simulink model "ResearchPaper4Fig8"  (R2015b)
settings: Solver=VariableStepAuto  StartTime=0.0  StopTime=10.0  RelTol=1e-3
libraries: xbsIndex_r4 x484, commfilt2 x1, commrandsrc3 x1, commdigbbndam3 x1
(part 3 of 3)

== system ResearchPaper4Fig8/Conventional RVTDNN6/Hidden Neuron4/Weight Update3 for H.N ==
  eta'grad : Inport
  xin1 : Inport  Port=2
  AddSub : xbsIndex_r4/AddSub  mode=Addition  use_carryin=off  use_carryout=off  en=off  latency=0  precision=Full  arith_type=Unsigned  n_bits=16  bin_pt=14  quantization=Truncate  overflow=Wrap  use_behavioral_HDL=off  hw_selection=Fabric  pipelined=off  dbl_ovrd=off  block_type=addsub
  Mult : xbsIndex_r4/Mult  precision=Full  arith_type="Signed  (2's comp)"  n_bits=16  bin_pt=14  quantization=Truncate  overflow=Wrap  en=off  latency=0  use_behavioral_HDL=off  opt=Speed  use_embedded=on  optimum_pipeline=off  pipeline=on  dbl_ovrd=off  use_rpm=on  placement_style=Triangular  block_type=mult
  Register : xbsIndex_r4/Register  init=0  rst=off  en=off  dbl_ovrd=off  block_type=register
  w11 : Outport
  wires:
  Mult/1 -> AddSub/1
  Register/1 -> w11/1, AddSub/2
  AddSub/1 -> Register/1
  eta'grad/1 -> Mult/1
  xin1/1 -> Mult/2

== system ResearchPaper4Fig8/Conventional RVTDNN6/Hidden Neuron4/Weight Update4 for H.N ==
  eta'grad : Inport
  xin1 : Inport  Port=2
  AddSub : xbsIndex_r4/AddSub  mode=Addition  use_carryin=off  use_carryout=off  en=off  latency=0  precision=Full  arith_type=Unsigned  n_bits=16  bin_pt=14  quantization=Truncate  overflow=Wrap  use_behavioral_HDL=off  hw_selection=Fabric  pipelined=off  dbl_ovrd=off  block_type=addsub
  Mult : xbsIndex_r4/Mult  precision=Full  arith_type="Signed  (2's comp)"  n_bits=16  bin_pt=14  quantization=Truncate  overflow=Wrap  en=off  latency=0  use_behavioral_HDL=off  opt=Speed  use_embedded=on  optimum_pipeline=off  pipeline=on  dbl_ovrd=off  use_rpm=on  placement_style=Triangular  block_type=mult
  Register : xbsIndex_r4/Register  init=0  rst=off  en=off  dbl_ovrd=off  block_type=register
  w11 : Outport
  wires:
  Mult/1 -> AddSub/1
  Register/1 -> w11/1, AddSub/2
  AddSub/1 -> Register/1
  eta'grad/1 -> Mult/1
  xin1/1 -> Mult/2

== system ResearchPaper4Fig8/Conventional RVTDNN6/Hidden Neuron4/Weight Update5 for H.N ==
  eta'grad : Inport
  xin1 : Inport  Port=2
  AddSub : xbsIndex_r4/AddSub  mode=Addition  use_carryin=off  use_carryout=off  en=off  latency=0  precision=Full  arith_type=Unsigned  n_bits=16  bin_pt=14  quantization=Truncate  overflow=Wrap  use_behavioral_HDL=off  hw_selection=Fabric  pipelined=off  dbl_ovrd=off  block_type=addsub
  Mult : xbsIndex_r4/Mult  precision=Full  arith_type="Signed  (2's comp)"  n_bits=16  bin_pt=14  quantization=Truncate  overflow=Wrap  en=off  latency=0  use_behavioral_HDL=off  opt=Speed  use_embedded=on  optimum_pipeline=off  pipeline=on  dbl_ovrd=off  use_rpm=on  placement_style=Triangular  block_type=mult
  Register : xbsIndex_r4/Register  init=0  rst=off  en=off  dbl_ovrd=off  block_type=register
  w11 : Outport
  wires:
  Mult/1 -> AddSub/1
  Register/1 -> w11/1, AddSub/2
  AddSub/1 -> Register/1
  eta'grad/1 -> Mult/1
  xin1/1 -> Mult/2

== system ResearchPaper4Fig8/Conventional RVTDNN6/Hidden Neuron4/Weight Update6 for H.N ==
  eta'grad : Inport
  xin1 : Inport  Port=2
  AddSub : xbsIndex_r4/AddSub  mode=Addition  use_carryin=off  use_carryout=off  en=off  latency=0  precision=Full  arith_type=Unsigned  n_bits=16  bin_pt=14  quantization=Truncate  overflow=Wrap  use_behavioral_HDL=off  hw_selection=Fabric  pipelined=off  dbl_ovrd=off  block_type=addsub
  Mult : xbsIndex_r4/Mult  precision=Full  arith_type="Signed  (2's comp)"  n_bits=16  bin_pt=14  quantization=Truncate  overflow=Wrap  en=off  latency=0  use_behavioral_HDL=off  opt=Speed  use_embedded=on  optimum_pipeline=off  pipeline=on  dbl_ovrd=off  use_rpm=on  placement_style=Triangular  block_type=mult
  Register : xbsIndex_r4/Register  init=0  rst=off  en=off  dbl_ovrd=off  block_type=register
  w11 : Outport
  wires:
  Mult/1 -> AddSub/1
  Register/1 -> w11/1, AddSub/2
  AddSub/1 -> Register/1
  eta'grad/1 -> Mult/1
  xin1/1 -> Mult/2

== system ResearchPaper4Fig8/Conventional RVTDNN6/Hidden Neuron5/Bias Update for H.N ==
  eta'grad : Inport
  AddSub : xbsIndex_r4/AddSub  mode=Addition  use_carryin=off  use_carryout=off  en=off  latency=0  precision=Full  arith_type=Unsigned  n_bits=16  bin_pt=14  quantization=Truncate  overflow=Wrap  use_behavioral_HDL=off  hw_selection=Fabric  pipelined=off  dbl_ovrd=off  block_type=addsub
  Register : xbsIndex_r4/Register  init=0  rst=off  en=off  dbl_ovrd=off  block_type=register
  w10 : Outport
  wires:
  Register/1 -> w10/1, AddSub/2
  AddSub/1 -> Register/1
  eta'grad/1 -> AddSub/1

== system ResearchPaper4Fig8/Conventional RVTDNN6/Hidden Neuron5/Hyperbolic Tangent ==
  In1 : Inport
  Constant : xbsIndex_r4/Constant  const=0.0  gui_display_data_type=Fixed-point  arith_type=Signed (2's comp)  n_bits=16  bin_pt=14  preci_type=Single  exp_width=8  frac_width=24  explicit_period=off  period=1  equ=P=C  opselect=C  inp2=PCIN>>17  opr=+  inp1=P  carry=CIN  dbl_ovrd=off  block_type=constant
  Mux : xbsIndex_r4/Mux  inputs=2  en=off  latency=0  precision=Full  arith_type=Unsigned  n_bits=16  bin_pt=14  quantization=Truncate  overflow=Wrap  dbl_ovrd=off  block_type=mux
  Mux1 : xbsIndex_r4/Mux  inputs=2  en=off  latency=0  precision=Full  arith_type=Unsigned  n_bits=16  bin_pt=14  quantization=Truncate  overflow=Wrap  dbl_ovrd=off  block_type=mux
  Negate : xbsIndex_r4/Negate  precision=Full  arith_type=Unsigned  n_bits=16  bin_pt=14  quantization=Truncate  overflow=Wrap  en=off  latency=0  dbl_ovrd=off  block_type=negate
  Negate1 : xbsIndex_r4/Negate  precision=Full  arith_type=Unsigned  n_bits=16  bin_pt=14  quantization=Truncate  overflow=Wrap  en=off  latency=0  dbl_ovrd=off  block_type=negate
  ROM : xbsIndex_r4/ROM  depth=16  initVector=sin(pi*(0:15)/16)  distributed_mem=Distributed memory  rst=off  init_reg=0  en=off  latency=0  gui_display_data_type=Fixed-point  arith_type="Signed  (2's comp)"  n_bits=16  bin_pt=14  preci_type=Single  exp_width=8  frac_width=24  optimize=Area  use_rpm=on  dbl_ovrd=off  block_type=sprom
  Relational : xbsIndex_r4/Relational  mode=a>b  op_type=Bool  en=off  latency=0  dbl_ovrd=off  block_type=relational
  Shift : xbsIndex_r4/Shift  shift_dir=Left  shift_bits=13  en=off  latency=0  precision=Full  arith_type="Signed  (2's comp)"  n_bits=16  bin_pt=14  quantization=Truncate  overflow=Wrap  dbl_ovrd=off  block_type=shift
  Out1 : Outport
  wires:
  Relational/1 -> Mux1/1, Mux/1
  Mux/1 -> Shift/1
  Mux1/1 -> Out1/1
  ROM/1 -> Negate1/1, Mux1/2
  Negate1/1 -> Mux1/3
  Constant/1 -> Relational/1
  In1/1 -> Negate/1, Relational/2, Mux/2
  Negate/1 -> Mux/3
  Shift/1 -> ROM/1

== system ResearchPaper4Fig8/Conventional RVTDNN6/Hidden Neuron5/Sum ==
  In1 : Inport
  In2 : Inport  Port=2
  In3 : Inport  Port=3
  In4 : Inport  Port=4
  In5 : Inport  Port=5
  In6 : Inport  Port=6
  In7 : Inport  Port=7
  AddSub{,1..5} (6 alike) : xbsIndex_r4/AddSub  mode=Addition  use_carryin=off  use_carryout=off  en=off  latency=0  precision=Full  arith_type=Unsigned  n_bits=16  bin_pt=14  quantization=Truncate  overflow=Wrap  use_behavioral_HDL=off  hw_selection=Fabric  pipelined=off  dbl_ovrd=off  block_type=addsub
  Out : Outport
  wires:
  AddSub4/1 -> AddSub5/2
  AddSub3/1 -> AddSub5/1
  In7/1 -> AddSub4/2
  AddSub1/1 -> AddSub3/2
  AddSub2/1 -> AddSub4/1
  In1/1 -> AddSub/1
  In6/1 -> AddSub2/2
  In2/1 -> AddSub/2
  In4/1 -> AddSub1/2
  AddSub/1 -> AddSub3/1
  In5/1 -> AddSub2/1
  AddSub5/1 -> Out/1
  In3/1 -> AddSub1/1

== system ResearchPaper4Fig8/Conventional RVTDNN6/Hidden Neuron5/Weight Update1 for H.N ==
  eta'grad : Inport
  xin1 : Inport  Port=2
  AddSub : xbsIndex_r4/AddSub  mode=Addition  use_carryin=off  use_carryout=off  en=off  latency=0  precision=Full  arith_type=Unsigned  n_bits=16  bin_pt=14  quantization=Truncate  overflow=Wrap  use_behavioral_HDL=off  hw_selection=Fabric  pipelined=off  dbl_ovrd=off  block_type=addsub
  Mult : xbsIndex_r4/Mult  precision=Full  arith_type="Signed  (2's comp)"  n_bits=16  bin_pt=14  quantization=Truncate  overflow=Wrap  en=off  latency=0  use_behavioral_HDL=off  opt=Speed  use_embedded=on  optimum_pipeline=off  pipeline=on  dbl_ovrd=off  use_rpm=on  placement_style=Triangular  block_type=mult
  Register : xbsIndex_r4/Register  init=0  rst=off  en=off  dbl_ovrd=off  block_type=register
  w11 : Outport
  wires:
  Mult/1 -> AddSub/1
  Register/1 -> w11/1, AddSub/2
  AddSub/1 -> Register/1
  eta'grad/1 -> Mult/1
  xin1/1 -> Mult/2

== system ResearchPaper4Fig8/Conventional RVTDNN6/Hidden Neuron5/Weight Update2 for H.N ==
  eta'grad : Inport
  xin1 : Inport  Port=2
  AddSub : xbsIndex_r4/AddSub  mode=Addition  use_carryin=off  use_carryout=off  en=off  latency=0  precision=Full  arith_type=Unsigned  n_bits=16  bin_pt=14  quantization=Truncate  overflow=Wrap  use_behavioral_HDL=off  hw_selection=Fabric  pipelined=off  dbl_ovrd=off  block_type=addsub
  Mult : xbsIndex_r4/Mult  precision=Full  arith_type="Signed  (2's comp)"  n_bits=16  bin_pt=14  quantization=Truncate  overflow=Wrap  en=off  latency=0  use_behavioral_HDL=off  opt=Speed  use_embedded=on  optimum_pipeline=off  pipeline=on  dbl_ovrd=off  use_rpm=on  placement_style=Triangular  block_type=mult
  Register : xbsIndex_r4/Register  init=0  rst=off  en=off  dbl_ovrd=off  block_type=register
  w11 : Outport
  wires:
  Mult/1 -> AddSub/1
  Register/1 -> w11/1, AddSub/2
  AddSub/1 -> Register/1
  eta'grad/1 -> Mult/1
  xin1/1 -> Mult/2

== system ResearchPaper4Fig8/Conventional RVTDNN6/Hidden Neuron5/Weight Update3 for H.N ==
  eta'grad : Inport
  xin1 : Inport  Port=2
  AddSub : xbsIndex_r4/AddSub  mode=Addition  use_carryin=off  use_carryout=off  en=off  latency=0  precision=Full  arith_type=Unsigned  n_bits=16  bin_pt=14  quantization=Truncate  overflow=Wrap  use_behavioral_HDL=off  hw_selection=Fabric  pipelined=off  dbl_ovrd=off  block_type=addsub
  Mult : xbsIndex_r4/Mult  precision=Full  arith_type="Signed  (2's comp)"  n_bits=16  bin_pt=14  quantization=Truncate  overflow=Wrap  en=off  latency=0  use_behavioral_HDL=off  opt=Speed  use_embedded=on  optimum_pipeline=off  pipeline=on  dbl_ovrd=off  use_rpm=on  placement_style=Triangular  block_type=mult
  Register : xbsIndex_r4/Register  init=0  rst=off  en=off  dbl_ovrd=off  block_type=register
  w11 : Outport
  wires:
  Mult/1 -> AddSub/1
  Register/1 -> w11/1, AddSub/2
  AddSub/1 -> Register/1
  eta'grad/1 -> Mult/1
  xin1/1 -> Mult/2

== system ResearchPaper4Fig8/Conventional RVTDNN6/Hidden Neuron5/Weight Update4 for H.N ==
  eta'grad : Inport
  xin1 : Inport  Port=2
  AddSub : xbsIndex_r4/AddSub  mode=Addition  use_carryin=off  use_carryout=off  en=off  latency=0  precision=Full  arith_type=Unsigned  n_bits=16  bin_pt=14  quantization=Truncate  overflow=Wrap  use_behavioral_HDL=off  hw_selection=Fabric  pipelined=off  dbl_ovrd=off  block_type=addsub
  Mult : xbsIndex_r4/Mult  precision=Full  arith_type="Signed  (2's comp)"  n_bits=16  bin_pt=14  quantization=Truncate  overflow=Wrap  en=off  latency=0  use_behavioral_HDL=off  opt=Speed  use_embedded=on  optimum_pipeline=off  pipeline=on  dbl_ovrd=off  use_rpm=on  placement_style=Triangular  block_type=mult
  Register : xbsIndex_r4/Register  init=0  rst=off  en=off  dbl_ovrd=off  block_type=register
  w11 : Outport
  wires:
  Mult/1 -> AddSub/1
  Register/1 -> w11/1, AddSub/2
  AddSub/1 -> Register/1
  eta'grad/1 -> Mult/1
  xin1/1 -> Mult/2

== system ResearchPaper4Fig8/Conventional RVTDNN6/Hidden Neuron5/Weight Update5 for H.N ==
  eta'grad : Inport
  xin1 : Inport  Port=2
  AddSub : xbsIndex_r4/AddSub  mode=Addition  use_carryin=off  use_carryout=off  en=off  latency=0  precision=Full  arith_type=Unsigned  n_bits=16  bin_pt=14  quantization=Truncate  overflow=Wrap  use_behavioral_HDL=off  hw_selection=Fabric  pipelined=off  dbl_ovrd=off  block_type=addsub
  Mult : xbsIndex_r4/Mult  precision=Full  arith_type="Signed  (2's comp)"  n_bits=16  bin_pt=14  quantization=Truncate  overflow=Wrap  en=off  latency=0  use_behavioral_HDL=off  opt=Speed  use_embedded=on  optimum_pipeline=off  pipeline=on  dbl_ovrd=off  use_rpm=on  placement_style=Triangular  block_type=mult
  Register : xbsIndex_r4/Register  init=0  rst=off  en=off  dbl_ovrd=off  block_type=register
  w11 : Outport
  wires:
  Mult/1 -> AddSub/1
  Register/1 -> w11/1, AddSub/2
  AddSub/1 -> Register/1
  eta'grad/1 -> Mult/1
  xin1/1 -> Mult/2

== system ResearchPaper4Fig8/Conventional RVTDNN6/Hidden Neuron5/Weight Update6 for H.N ==
  eta'grad : Inport
  xin1 : Inport  Port=2
  AddSub : xbsIndex_r4/AddSub  mode=Addition  use_carryin=off  use_carryout=off  en=off  latency=0  precision=Full  arith_type=Unsigned  n_bits=16  bin_pt=14  quantization=Truncate  overflow=Wrap  use_behavioral_HDL=off  hw_selection=Fabric  pipelined=off  dbl_ovrd=off  block_type=addsub
  Mult : xbsIndex_r4/Mult  precision=Full  arith_type="Signed  (2's comp)"  n_bits=16  bin_pt=14  quantization=Truncate  overflow=Wrap  en=off  latency=0  use_behavioral_HDL=off  opt=Speed  use_embedded=on  optimum_pipeline=off  pipeline=on  dbl_ovrd=off  use_rpm=on  placement_style=Triangular  block_type=mult
  Register : xbsIndex_r4/Register  init=0  rst=off  en=off  dbl_ovrd=off  block_type=register
  w11 : Outport
  wires:
  Mult/1 -> AddSub/1
  Register/1 -> w11/1, AddSub/2
  AddSub/1 -> Register/1
  eta'grad/1 -> Mult/1
  xin1/1 -> Mult/2

== system ResearchPaper4Fig8/Conventional RVTDNN6/Hidden Neuron6/Bias Update for H.N ==
  eta'grad : Inport
  AddSub : xbsIndex_r4/AddSub  mode=Addition  use_carryin=off  use_carryout=off  en=off  latency=0  precision=Full  arith_type=Unsigned  n_bits=16  bin_pt=14  quantization=Truncate  overflow=Wrap  use_behavioral_HDL=off  hw_selection=Fabric  pipelined=off  dbl_ovrd=off  block_type=addsub
  Register : xbsIndex_r4/Register  init=0  rst=off  en=off  dbl_ovrd=off  block_type=register
  w10 : Outport
  wires:
  Register/1 -> w10/1, AddSub/2
  AddSub/1 -> Register/1
  eta'grad/1 -> AddSub/1

== system ResearchPaper4Fig8/Conventional RVTDNN6/Hidden Neuron6/Hyperbolic Tangent ==
  In1 : Inport
  Constant : xbsIndex_r4/Constant  const=0.0  gui_display_data_type=Fixed-point  arith_type=Signed (2's comp)  n_bits=16  bin_pt=14  preci_type=Single  exp_width=8  frac_width=24  explicit_period=off  period=1  equ=P=C  opselect=C  inp2=PCIN>>17  opr=+  inp1=P  carry=CIN  dbl_ovrd=off  block_type=constant
  Mux : xbsIndex_r4/Mux  inputs=2  en=off  latency=0  precision=Full  arith_type=Unsigned  n_bits=16  bin_pt=14  quantization=Truncate  overflow=Wrap  dbl_ovrd=off  block_type=mux
  Mux1 : xbsIndex_r4/Mux  inputs=2  en=off  latency=0  precision=Full  arith_type=Unsigned  n_bits=16  bin_pt=14  quantization=Truncate  overflow=Wrap  dbl_ovrd=off  block_type=mux
  Negate : xbsIndex_r4/Negate  precision=Full  arith_type=Unsigned  n_bits=16  bin_pt=14  quantization=Truncate  overflow=Wrap  en=off  latency=0  dbl_ovrd=off  block_type=negate
  Negate1 : xbsIndex_r4/Negate  precision=Full  arith_type=Unsigned  n_bits=16  bin_pt=14  quantization=Truncate  overflow=Wrap  en=off  latency=0  dbl_ovrd=off  block_type=negate
  ROM : xbsIndex_r4/ROM  depth=16  initVector=sin(pi*(0:15)/16)  distributed_mem=Distributed memory  rst=off  init_reg=0  en=off  latency=0  gui_display_data_type=Fixed-point  arith_type="Signed  (2's comp)"  n_bits=16  bin_pt=14  preci_type=Single  exp_width=8  frac_width=24  optimize=Area  use_rpm=on  dbl_ovrd=off  block_type=sprom
  Relational : xbsIndex_r4/Relational  mode=a>b  op_type=Bool  en=off  latency=0  dbl_ovrd=off  block_type=relational
  Shift : xbsIndex_r4/Shift  shift_dir=Left  shift_bits=13  en=off  latency=0  precision=Full  arith_type="Signed  (2's comp)"  n_bits=16  bin_pt=14  quantization=Truncate  overflow=Wrap  dbl_ovrd=off  block_type=shift
  Out1 : Outport
  wires:
  Relational/1 -> Mux1/1, Mux/1
  Mux/1 -> Shift/1
  Mux1/1 -> Out1/1
  ROM/1 -> Negate1/1, Mux1/2
  Negate1/1 -> Mux1/3
  Constant/1 -> Relational/1
  In1/1 -> Negate/1, Relational/2, Mux/2
  Negate/1 -> Mux/3
  Shift/1 -> ROM/1

== system ResearchPaper4Fig8/Conventional RVTDNN6/Hidden Neuron6/Sum ==
  In1 : Inport
  In2 : Inport  Port=2
  In3 : Inport  Port=3
  In4 : Inport  Port=4
  In5 : Inport  Port=5
  In6 : Inport  Port=6
  In7 : Inport  Port=7
  AddSub{,1..5} (6 alike) : xbsIndex_r4/AddSub  mode=Addition  use_carryin=off  use_carryout=off  en=off  latency=0  precision=Full  arith_type=Unsigned  n_bits=16  bin_pt=14  quantization=Truncate  overflow=Wrap  use_behavioral_HDL=off  hw_selection=Fabric  pipelined=off  dbl_ovrd=off  block_type=addsub
  Out : Outport
  wires:
  AddSub4/1 -> AddSub5/2
  AddSub3/1 -> AddSub5/1
  In7/1 -> AddSub4/2
  AddSub1/1 -> AddSub3/2
  AddSub2/1 -> AddSub4/1
  In1/1 -> AddSub/1
  In6/1 -> AddSub2/2
  In2/1 -> AddSub/2
  In4/1 -> AddSub1/2
  AddSub/1 -> AddSub3/1
  In5/1 -> AddSub2/1
  AddSub5/1 -> Out/1
  In3/1 -> AddSub1/1

== system ResearchPaper4Fig8/Conventional RVTDNN6/Hidden Neuron6/Weight Update1 for H.N ==
  eta'grad : Inport
  xin1 : Inport  Port=2
  AddSub : xbsIndex_r4/AddSub  mode=Addition  use_carryin=off  use_carryout=off  en=off  latency=0  precision=Full  arith_type=Unsigned  n_bits=16  bin_pt=14  quantization=Truncate  overflow=Wrap  use_behavioral_HDL=off  hw_selection=Fabric  pipelined=off  dbl_ovrd=off  block_type=addsub
  Mult : xbsIndex_r4/Mult  precision=Full  arith_type="Signed  (2's comp)"  n_bits=16  bin_pt=14  quantization=Truncate  overflow=Wrap  en=off  latency=0  use_behavioral_HDL=off  opt=Speed  use_embedded=on  optimum_pipeline=off  pipeline=on  dbl_ovrd=off  use_rpm=on  placement_style=Triangular  block_type=mult
  Register : xbsIndex_r4/Register  init=0  rst=off  en=off  dbl_ovrd=off  block_type=register
  w11 : Outport
  wires:
  Mult/1 -> AddSub/1
  Register/1 -> w11/1, AddSub/2
  AddSub/1 -> Register/1
  eta'grad/1 -> Mult/1
  xin1/1 -> Mult/2

== system ResearchPaper4Fig8/Conventional RVTDNN6/Hidden Neuron6/Weight Update2 for H.N ==
  eta'grad : Inport
  xin1 : Inport  Port=2
  AddSub : xbsIndex_r4/AddSub  mode=Addition  use_carryin=off  use_carryout=off  en=off  latency=0  precision=Full  arith_type=Unsigned  n_bits=16  bin_pt=14  quantization=Truncate  overflow=Wrap  use_behavioral_HDL=off  hw_selection=Fabric  pipelined=off  dbl_ovrd=off  block_type=addsub
  Mult : xbsIndex_r4/Mult  precision=Full  arith_type="Signed  (2's comp)"  n_bits=16  bin_pt=14  quantization=Truncate  overflow=Wrap  en=off  latency=0  use_behavioral_HDL=off  opt=Speed  use_embedded=on  optimum_pipeline=off  pipeline=on  dbl_ovrd=off  use_rpm=on  placement_style=Triangular  block_type=mult
  Register : xbsIndex_r4/Register  init=0  rst=off  en=off  dbl_ovrd=off  block_type=register
  w11 : Outport
  wires:
  Mult/1 -> AddSub/1
  Register/1 -> w11/1, AddSub/2
  AddSub/1 -> Register/1
  eta'grad/1 -> Mult/1
  xin1/1 -> Mult/2

== system ResearchPaper4Fig8/Conventional RVTDNN6/Hidden Neuron6/Weight Update3 for H.N ==
  eta'grad : Inport
  xin1 : Inport  Port=2
  AddSub : xbsIndex_r4/AddSub  mode=Addition  use_carryin=off  use_carryout=off  en=off  latency=0  precision=Full  arith_type=Unsigned  n_bits=16  bin_pt=14  quantization=Truncate  overflow=Wrap  use_behavioral_HDL=off  hw_selection=Fabric  pipelined=off  dbl_ovrd=off  block_type=addsub
  Mult : xbsIndex_r4/Mult  precision=Full  arith_type="Signed  (2's comp)"  n_bits=16  bin_pt=14  quantization=Truncate  overflow=Wrap  en=off  latency=0  use_behavioral_HDL=off  opt=Speed  use_embedded=on  optimum_pipeline=off  pipeline=on  dbl_ovrd=off  use_rpm=on  placement_style=Triangular  block_type=mult
  Register : xbsIndex_r4/Register  init=0  rst=off  en=off  dbl_ovrd=off  block_type=register
  w11 : Outport
  wires:
  Mult/1 -> AddSub/1
  Register/1 -> w11/1, AddSub/2
  AddSub/1 -> Register/1
  eta'grad/1 -> Mult/1
  xin1/1 -> Mult/2

== system ResearchPaper4Fig8/Conventional RVTDNN6/Hidden Neuron6/Weight Update4 for H.N ==
  eta'grad : Inport
  xin1 : Inport  Port=2
  AddSub : xbsIndex_r4/AddSub  mode=Addition  use_carryin=off  use_carryout=off  en=off  latency=0  precision=Full  arith_type=Unsigned  n_bits=16  bin_pt=14  quantization=Truncate  overflow=Wrap  use_behavioral_HDL=off  hw_selection=Fabric  pipelined=off  dbl_ovrd=off  block_type=addsub
  Mult : xbsIndex_r4/Mult  precision=Full  arith_type="Signed  (2's comp)"  n_bits=16  bin_pt=14  quantization=Truncate  overflow=Wrap  en=off  latency=0  use_behavioral_HDL=off  opt=Speed  use_embedded=on  optimum_pipeline=off  pipeline=on  dbl_ovrd=off  use_rpm=on  placement_style=Triangular  block_type=mult
  Register : xbsIndex_r4/Register  init=0  rst=off  en=off  dbl_ovrd=off  block_type=register
  w11 : Outport
  wires:
  Mult/1 -> AddSub/1
  Register/1 -> w11/1, AddSub/2
  AddSub/1 -> Register/1
  eta'grad/1 -> Mult/1
  xin1/1 -> Mult/2

== system ResearchPaper4Fig8/Conventional RVTDNN6/Hidden Neuron6/Weight Update5 for H.N ==
  eta'grad : Inport
  xin1 : Inport  Port=2
  AddSub : xbsIndex_r4/AddSub  mode=Addition  use_carryin=off  use_carryout=off  en=off  latency=0  precision=Full  arith_type=Unsigned  n_bits=16  bin_pt=14  quantization=Truncate  overflow=Wrap  use_behavioral_HDL=off  hw_selection=Fabric  pipelined=off  dbl_ovrd=off  block_type=addsub
  Mult : xbsIndex_r4/Mult  precision=Full  arith_type="Signed  (2's comp)"  n_bits=16  bin_pt=14  quantization=Truncate  overflow=Wrap  en=off  latency=0  use_behavioral_HDL=off  opt=Speed  use_embedded=on  optimum_pipeline=off  pipeline=on  dbl_ovrd=off  use_rpm=on  placement_style=Triangular  block_type=mult
  Register : xbsIndex_r4/Register  init=0  rst=off  en=off  dbl_ovrd=off  block_type=register
  w11 : Outport
  wires:
  Mult/1 -> AddSub/1
  Register/1 -> w11/1, AddSub/2
  AddSub/1 -> Register/1
  eta'grad/1 -> Mult/1
  xin1/1 -> Mult/2

== system ResearchPaper4Fig8/Conventional RVTDNN6/Hidden Neuron6/Weight Update6 for H.N ==
  eta'grad : Inport
  xin1 : Inport  Port=2
  AddSub : xbsIndex_r4/AddSub  mode=Addition  use_carryin=off  use_carryout=off  en=off  latency=0  precision=Full  arith_type=Unsigned  n_bits=16  bin_pt=14  quantization=Truncate  overflow=Wrap  use_behavioral_HDL=off  hw_selection=Fabric  pipelined=off  dbl_ovrd=off  block_type=addsub
  Mult : xbsIndex_r4/Mult  precision=Full  arith_type="Signed  (2's comp)"  n_bits=16  bin_pt=14  quantization=Truncate  overflow=Wrap  en=off  latency=0  use_behavioral_HDL=off  opt=Speed  use_embedded=on  optimum_pipeline=off  pipeline=on  dbl_ovrd=off  use_rpm=on  placement_style=Triangular  block_type=mult
  Register : xbsIndex_r4/Register  init=0  rst=off  en=off  dbl_ovrd=off  block_type=register
  w11 : Outport
  wires:
  Mult/1 -> AddSub/1
  Register/1 -> w11/1, AddSub/2
  AddSub/1 -> Register/1
  eta'grad/1 -> Mult/1
  xin1/1 -> Mult/2

== system ResearchPaper4Fig8/Conventional RVTDNN6/Output Neuron1/Bias Update for O.N ==
  grad : Inport
  AddSub : xbsIndex_r4/AddSub  mode=Addition  use_carryin=off  use_carryout=off  en=off  latency=0  precision=Full  arith_type=Unsigned  n_bits=16  bin_pt=14  quantization=Truncate  overflow=Wrap  use_behavioral_HDL=off  hw_selection=Fabric  pipelined=off  dbl_ovrd=off  block_type=addsub
  Register : xbsIndex_r4/Register  init=0  rst=off  en=off  dbl_ovrd=off  block_type=register
  w10 : Outport
  wires:
  Register/1 -> w10/1, AddSub/2
  AddSub/1 -> Register/1
  grad/1 -> AddSub/1

== system ResearchPaper4Fig8/Conventional RVTDNN6/Output Neuron1/Sum ==
  In1 : Inport
  In2 : Inport  Port=2
  In3 : Inport  Port=3
  In4 : Inport  Port=4
  In5 : Inport  Port=5
  In6 : Inport  Port=6
  In7 : Inport  Port=7
  AddSub{,1..5} (6 alike) : xbsIndex_r4/AddSub  mode=Addition  use_carryin=off  use_carryout=off  en=off  latency=0  precision=Full  arith_type=Unsigned  n_bits=16  bin_pt=14  quantization=Truncate  overflow=Wrap  use_behavioral_HDL=off  hw_selection=Fabric  pipelined=off  dbl_ovrd=off  block_type=addsub
  Out : Outport
  wires:
  AddSub4/1 -> AddSub5/2
  AddSub3/1 -> AddSub5/1
  In7/1 -> AddSub4/2
  AddSub1/1 -> AddSub3/2
  AddSub2/1 -> AddSub4/1
  In1/1 -> AddSub/1
  In6/1 -> AddSub2/2
  In2/1 -> AddSub/2
  In4/1 -> AddSub1/2
  AddSub/1 -> AddSub3/1
  In5/1 -> AddSub2/1
  AddSub5/1 -> Out/1
  In3/1 -> AddSub1/1

== system ResearchPaper4Fig8/Conventional RVTDNN6/Output Neuron1/Weight Update1 for O.N ==
  eta'grad : Inport
  o1 : Inport  Port=2
  AddSub : xbsIndex_r4/AddSub  mode=Addition  use_carryin=off  use_carryout=off  en=off  latency=0  precision=Full  arith_type=Unsigned  n_bits=16  bin_pt=14  quantization=Truncate  overflow=Wrap  use_behavioral_HDL=off  hw_selection=Fabric  pipelined=off  dbl_ovrd=off  block_type=addsub
  Mult : xbsIndex_r4/Mult  precision=Full  arith_type="Signed  (2's comp)"  n_bits=16  bin_pt=14  quantization=Truncate  overflow=Wrap  en=off  latency=0  use_behavioral_HDL=off  opt=Speed  use_embedded=on  optimum_pipeline=off  pipeline=on  dbl_ovrd=off  use_rpm=on  placement_style=Triangular  block_type=mult
  Register : xbsIndex_r4/Register  init=0  rst=off  en=off  dbl_ovrd=off  block_type=register
  w11 : Outport
  wires:
  Mult/1 -> AddSub/1
  Register/1 -> w11/1, AddSub/2
  AddSub/1 -> Register/1
  eta'grad/1 -> Mult/1
  o1/1 -> Mult/2

== system ResearchPaper4Fig8/Conventional RVTDNN6/Output Neuron1/Weight Update2 for O.N ==
  eta'grad : Inport
  o1 : Inport  Port=2
  AddSub : xbsIndex_r4/AddSub  mode=Addition  use_carryin=off  use_carryout=off  en=off  latency=0  precision=Full  arith_type=Unsigned  n_bits=16  bin_pt=14  quantization=Truncate  overflow=Wrap  use_behavioral_HDL=off  hw_selection=Fabric  pipelined=off  dbl_ovrd=off  block_type=addsub
  Mult : xbsIndex_r4/Mult  precision=Full  arith_type="Signed  (2's comp)"  n_bits=16  bin_pt=14  quantization=Truncate  overflow=Wrap  en=off  latency=0  use_behavioral_HDL=off  opt=Speed  use_embedded=on  optimum_pipeline=off  pipeline=on  dbl_ovrd=off  use_rpm=on  placement_style=Triangular  block_type=mult
  Register : xbsIndex_r4/Register  init=0  rst=off  en=off  dbl_ovrd=off  block_type=register
  w11 : Outport
  wires:
  Mult/1 -> AddSub/1
  Register/1 -> w11/1, AddSub/2
  AddSub/1 -> Register/1
  eta'grad/1 -> Mult/1
  o1/1 -> Mult/2

== system ResearchPaper4Fig8/Conventional RVTDNN6/Output Neuron1/Weight Update3 for O.N ==
  eta'grad : Inport
  o1 : Inport  Port=2
  AddSub : xbsIndex_r4/AddSub  mode=Addition  use_carryin=off  use_carryout=off  en=off  latency=0  precision=Full  arith_type=Unsigned  n_bits=16  bin_pt=14  quantization=Truncate  overflow=Wrap  use_behavioral_HDL=off  hw_selection=Fabric  pipelined=off  dbl_ovrd=off  block_type=addsub
  Mult : xbsIndex_r4/Mult  precision=Full  arith_type="Signed  (2's comp)"  n_bits=16  bin_pt=14  quantization=Truncate  overflow=Wrap  en=off  latency=0  use_behavioral_HDL=off  opt=Speed  use_embedded=on  optimum_pipeline=off  pipeline=on  dbl_ovrd=off  use_rpm=on  placement_style=Triangular  block_type=mult
  Register : xbsIndex_r4/Register  init=0  rst=off  en=off  dbl_ovrd=off  block_type=register
  w11 : Outport
  wires:
  Mult/1 -> AddSub/1
  Register/1 -> w11/1, AddSub/2
  AddSub/1 -> Register/1
  eta'grad/1 -> Mult/1
  o1/1 -> Mult/2

== system ResearchPaper4Fig8/Conventional RVTDNN6/Output Neuron1/Weight Update4 for O.N ==
  eta'grad : Inport
  o1 : Inport  Port=2
  AddSub : xbsIndex_r4/AddSub  mode=Addition  use_carryin=off  use_carryout=off  en=off  latency=0  precision=Full  arith_type=Unsigned  n_bits=16  bin_pt=14  quantization=Truncate  overflow=Wrap  use_behavioral_HDL=off  hw_selection=Fabric  pipelined=off  dbl_ovrd=off  block_type=addsub
  Mult : xbsIndex_r4/Mult  precision=Full  arith_type="Signed  (2's comp)"  n_bits=16  bin_pt=14  quantization=Truncate  overflow=Wrap  en=off  latency=0  use_behavioral_HDL=off  opt=Speed  use_embedded=on  optimum_pipeline=off  pipeline=on  dbl_ovrd=off  use_rpm=on  placement_style=Triangular  block_type=mult
  Register : xbsIndex_r4/Register  init=0  rst=off  en=off  dbl_ovrd=off  block_type=register
  w11 : Outport
  wires:
  Mult/1 -> AddSub/1
  Register/1 -> w11/1, AddSub/2
  AddSub/1 -> Register/1
  eta'grad/1 -> Mult/1
  o1/1 -> Mult/2

== system ResearchPaper4Fig8/Conventional RVTDNN6/Output Neuron1/Weight Update5 for O.N ==
  eta'grad : Inport
  o1 : Inport  Port=2
  AddSub : xbsIndex_r4/AddSub  mode=Addition  use_carryin=off  use_carryout=off  en=off  latency=0  precision=Full  arith_type=Unsigned  n_bits=16  bin_pt=14  quantization=Truncate  overflow=Wrap  use_behavioral_HDL=off  hw_selection=Fabric  pipelined=off  dbl_ovrd=off  block_type=addsub
  Mult : xbsIndex_r4/Mult  precision=Full  arith_type="Signed  (2's comp)"  n_bits=16  bin_pt=14  quantization=Truncate  overflow=Wrap  en=off  latency=0  use_behavioral_HDL=off  opt=Speed  use_embedded=on  optimum_pipeline=off  pipeline=on  dbl_ovrd=off  use_rpm=on  placement_style=Triangular  block_type=mult
  Register : xbsIndex_r4/Register  init=0  rst=off  en=off  dbl_ovrd=off  block_type=register
  w11 : Outport
  wires:
  Mult/1 -> AddSub/1
  Register/1 -> w11/1, AddSub/2
  AddSub/1 -> Register/1
  eta'grad/1 -> Mult/1
  o1/1 -> Mult/2

== system ResearchPaper4Fig8/Conventional RVTDNN6/Output Neuron1/Weight Update6 for O.N ==
  eta'grad : Inport
  o1 : Inport  Port=2
  AddSub : xbsIndex_r4/AddSub  mode=Addition  use_carryin=off  use_carryout=off  en=off  latency=0  precision=Full  arith_type=Unsigned  n_bits=16  bin_pt=14  quantization=Truncate  overflow=Wrap  use_behavioral_HDL=off  hw_selection=Fabric  pipelined=off  dbl_ovrd=off  block_type=addsub
  Mult : xbsIndex_r4/Mult  precision=Full  arith_type="Signed  (2's comp)"  n_bits=16  bin_pt=14  quantization=Truncate  overflow=Wrap  en=off  latency=0  use_behavioral_HDL=off  opt=Speed  use_embedded=on  optimum_pipeline=off  pipeline=on  dbl_ovrd=off  use_rpm=on  placement_style=Triangular  block_type=mult
  Register : xbsIndex_r4/Register  init=0  rst=off  en=off  dbl_ovrd=off  block_type=register
  w11 : Outport
  wires:
  Mult/1 -> AddSub/1
  Register/1 -> w11/1, AddSub/2
  AddSub/1 -> Register/1
  eta'grad/1 -> Mult/1
  o1/1 -> Mult/2

== system ResearchPaper4Fig8/Conventional RVTDNN6/Output Neuron2/Bias Update for O.N ==
  grad : Inport
  AddSub : xbsIndex_r4/AddSub  mode=Addition  use_carryin=off  use_carryout=off  en=off  latency=0  precision=Full  arith_type=Unsigned  n_bits=16  bin_pt=14  quantization=Truncate  overflow=Wrap  use_behavioral_HDL=off  hw_selection=Fabric  pipelined=off  dbl_ovrd=off  block_type=addsub
  Register : xbsIndex_r4/Register  init=0  rst=off  en=off  dbl_ovrd=off  block_type=register
  w10 : Outport
  wires:
  Register/1 -> w10/1, AddSub/2
  AddSub/1 -> Register/1
  grad/1 -> AddSub/1

== system ResearchPaper4Fig8/Conventional RVTDNN6/Output Neuron2/Sum ==
  In1 : Inport
  In2 : Inport  Port=2
  In3 : Inport  Port=3
  In4 : Inport  Port=4
  In5 : Inport  Port=5
  In6 : Inport  Port=6
  In7 : Inport  Port=7
  AddSub{,1..5} (6 alike) : xbsIndex_r4/AddSub  mode=Addition  use_carryin=off  use_carryout=off  en=off  latency=0  precision=Full  arith_type=Unsigned  n_bits=16  bin_pt=14  quantization=Truncate  overflow=Wrap  use_behavioral_HDL=off  hw_selection=Fabric  pipelined=off  dbl_ovrd=off  block_type=addsub
  Out : Outport
  wires:
  AddSub4/1 -> AddSub5/2
  AddSub3/1 -> AddSub5/1
  In7/1 -> AddSub4/2
  AddSub1/1 -> AddSub3/2
  AddSub2/1 -> AddSub4/1
  In1/1 -> AddSub/1
  In6/1 -> AddSub2/2
  In2/1 -> AddSub/2
  In4/1 -> AddSub1/2
  AddSub/1 -> AddSub3/1
  In5/1 -> AddSub2/1
  AddSub5/1 -> Out/1
  In3/1 -> AddSub1/1

== system ResearchPaper4Fig8/Conventional RVTDNN6/Output Neuron2/Weight Update1 for O.N ==
  eta'grad : Inport
  o1 : Inport  Port=2
  AddSub : xbsIndex_r4/AddSub  mode=Addition  use_carryin=off  use_carryout=off  en=off  latency=0  precision=Full  arith_type=Unsigned  n_bits=16  bin_pt=14  quantization=Truncate  overflow=Wrap  use_behavioral_HDL=off  hw_selection=Fabric  pipelined=off  dbl_ovrd=off  block_type=addsub
  Mult : xbsIndex_r4/Mult  precision=Full  arith_type="Signed  (2's comp)"  n_bits=16  bin_pt=14  quantization=Truncate  overflow=Wrap  en=off  latency=0  use_behavioral_HDL=off  opt=Speed  use_embedded=on  optimum_pipeline=off  pipeline=on  dbl_ovrd=off  use_rpm=on  placement_style=Triangular  block_type=mult
  Register : xbsIndex_r4/Register  init=0  rst=off  en=off  dbl_ovrd=off  block_type=register
  w11 : Outport
  wires:
  Mult/1 -> AddSub/1
  Register/1 -> w11/1, AddSub/2
  AddSub/1 -> Register/1
  eta'grad/1 -> Mult/1
  o1/1 -> Mult/2

== system ResearchPaper4Fig8/Conventional RVTDNN6/Output Neuron2/Weight Update2 for O.N ==
  eta'grad : Inport
  o1 : Inport  Port=2
  AddSub : xbsIndex_r4/AddSub  mode=Addition  use_carryin=off  use_carryout=off  en=off  latency=0  precision=Full  arith_type=Unsigned  n_bits=16  bin_pt=14  quantization=Truncate  overflow=Wrap  use_behavioral_HDL=off  hw_selection=Fabric  pipelined=off  dbl_ovrd=off  block_type=addsub
  Mult : xbsIndex_r4/Mult  precision=Full  arith_type="Signed  (2's comp)"  n_bits=16  bin_pt=14  quantization=Truncate  overflow=Wrap  en=off  latency=0  use_behavioral_HDL=off  opt=Speed  use_embedded=on  optimum_pipeline=off  pipeline=on  dbl_ovrd=off  use_rpm=on  placement_style=Triangular  block_type=mult
  Register : xbsIndex_r4/Register  init=0  rst=off  en=off  dbl_ovrd=off  block_type=register
  w11 : Outport
  wires:
  Mult/1 -> AddSub/1
  Register/1 -> w11/1, AddSub/2
  AddSub/1 -> Register/1
  eta'grad/1 -> Mult/1
  o1/1 -> Mult/2

== system ResearchPaper4Fig8/Conventional RVTDNN6/Output Neuron2/Weight Update3 for O.N ==
  eta'grad : Inport
  o1 : Inport  Port=2
  AddSub : xbsIndex_r4/AddSub  mode=Addition  use_carryin=off  use_carryout=off  en=off  latency=0  precision=Full  arith_type=Unsigned  n_bits=16  bin_pt=14  quantization=Truncate  overflow=Wrap  use_behavioral_HDL=off  hw_selection=Fabric  pipelined=off  dbl_ovrd=off  block_type=addsub
  Mult : xbsIndex_r4/Mult  precision=Full  arith_type="Signed  (2's comp)"  n_bits=16  bin_pt=14  quantization=Truncate  overflow=Wrap  en=off  latency=0  use_behavioral_HDL=off  opt=Speed  use_embedded=on  optimum_pipeline=off  pipeline=on  dbl_ovrd=off  use_rpm=on  placement_style=Triangular  block_type=mult
  Register : xbsIndex_r4/Register  init=0  rst=off  en=off  dbl_ovrd=off  block_type=register
  w11 : Outport
  wires:
  Mult/1 -> AddSub/1
  Register/1 -> w11/1, AddSub/2
  AddSub/1 -> Register/1
  eta'grad/1 -> Mult/1
  o1/1 -> Mult/2

== system ResearchPaper4Fig8/Conventional RVTDNN6/Output Neuron2/Weight Update4 for O.N ==
  eta'grad : Inport
  o1 : Inport  Port=2
  AddSub : xbsIndex_r4/AddSub  mode=Addition  use_carryin=off  use_carryout=off  en=off  latency=0  precision=Full  arith_type=Unsigned  n_bits=16  bin_pt=14  quantization=Truncate  overflow=Wrap  use_behavioral_HDL=off  hw_selection=Fabric  pipelined=off  dbl_ovrd=off  block_type=addsub
  Mult : xbsIndex_r4/Mult  precision=Full  arith_type="Signed  (2's comp)"  n_bits=16  bin_pt=14  quantization=Truncate  overflow=Wrap  en=off  latency=0  use_behavioral_HDL=off  opt=Speed  use_embedded=on  optimum_pipeline=off  pipeline=on  dbl_ovrd=off  use_rpm=on  placement_style=Triangular  block_type=mult
  Register : xbsIndex_r4/Register  init=0  rst=off  en=off  dbl_ovrd=off  block_type=register
  w11 : Outport
  wires:
  Mult/1 -> AddSub/1
  Register/1 -> w11/1, AddSub/2
  AddSub/1 -> Register/1
  eta'grad/1 -> Mult/1
  o1/1 -> Mult/2

== system ResearchPaper4Fig8/Conventional RVTDNN6/Output Neuron2/Weight Update5 for O.N ==
  eta'grad : Inport
  o1 : Inport  Port=2
  AddSub : xbsIndex_r4/AddSub  mode=Addition  use_carryin=off  use_carryout=off  en=off  latency=0  precision=Full  arith_type=Unsigned  n_bits=16  bin_pt=14  quantization=Truncate  overflow=Wrap  use_behavioral_HDL=off  hw_selection=Fabric  pipelined=off  dbl_ovrd=off  block_type=addsub
  Mult : xbsIndex_r4/Mult  precision=Full  arith_type="Signed  (2's comp)"  n_bits=16  bin_pt=14  quantization=Truncate  overflow=Wrap  en=off  latency=0  use_behavioral_HDL=off  opt=Speed  use_embedded=on  optimum_pipeline=off  pipeline=on  dbl_ovrd=off  use_rpm=on  placement_style=Triangular  block_type=mult
  Register : xbsIndex_r4/Register  init=0  rst=off  en=off  dbl_ovrd=off  block_type=register
  w11 : Outport
  wires:
  Mult/1 -> AddSub/1
  Register/1 -> w11/1, AddSub/2
  AddSub/1 -> Register/1
  eta'grad/1 -> Mult/1
  o1/1 -> Mult/2

== system ResearchPaper4Fig8/Conventional RVTDNN6/Output Neuron2/Weight Update6 for O.N ==
  eta'grad : Inport
  o1 : Inport  Port=2
  AddSub : xbsIndex_r4/AddSub  mode=Addition  use_carryin=off  use_carryout=off  en=off  latency=0  precision=Full  arith_type=Unsigned  n_bits=16  bin_pt=14  quantization=Truncate  overflow=Wrap  use_behavioral_HDL=off  hw_selection=Fabric  pipelined=off  dbl_ovrd=off  block_type=addsub
  Mult : xbsIndex_r4/Mult  precision=Full  arith_type="Signed  (2's comp)"  n_bits=16  bin_pt=14  quantization=Truncate  overflow=Wrap  en=off  latency=0  use_behavioral_HDL=off  opt=Speed  use_embedded=on  optimum_pipeline=off  pipeline=on  dbl_ovrd=off  use_rpm=on  placement_style=Triangular  block_type=mult
  Register : xbsIndex_r4/Register  init=0  rst=off  en=off  dbl_ovrd=off  block_type=register
  w11 : Outport
  wires:
  Mult/1 -> AddSub/1
  Register/1 -> w11/1, AddSub/2
  AddSub/1 -> Register/1
  eta'grad/1 -> Mult/1
  o1/1 -> Mult/2
